simulink model "Speed_Density"  (R2025b)
settings: Solver=VariableStepAuto  StartTime=0.0  StopTime=10.0  RelTol=1e-3
model workspace (MAT data in the model file):
  P0 = 1
  R_EGR = 1
  T0 = 1
  d0 = 1
  nv = 1
settings Model: Creator=Pai  LastModifiedBy=Pai

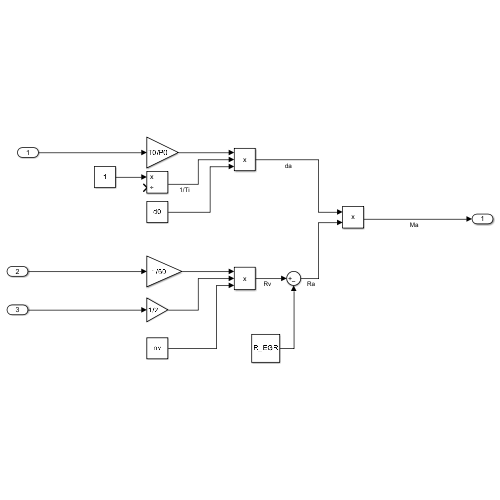
[thumbnail: Simulink's stored preview of the top-level diagram]
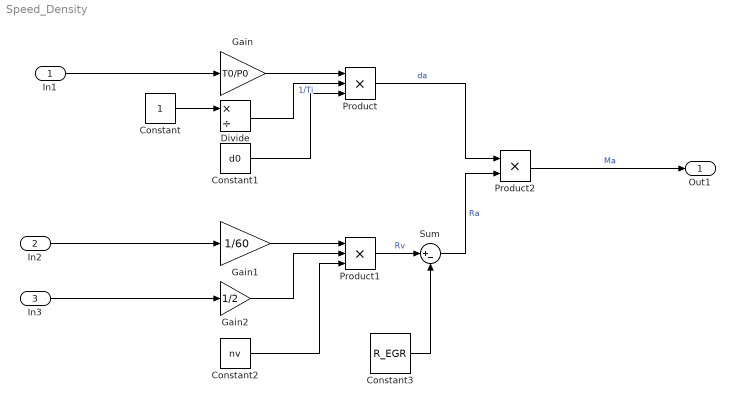
== system Speed_Density ==
  In1 : Inport
  In2 : Inport  Port=2
  In3 : Inport  Port=3
  Constant : Constant
  Constant1 : Constant  Value=d0
  Constant2 : Constant  Value=nv
  Constant3 : Constant  Value=R_EGR
  Divide : Product  Inputs=*/
  Gain : Gain  Gain=T0/P0
  Gain1 : Gain  Gain=1/60
  Gain2 : Gain  Gain=1/2
  Product : Product  Inputs=3
  Product1 : Product  Inputs=3
  Product2 : Product
  Sum : Sum  Inputs=|+-
  Out1 : Outport
  wires:
  Constant/1 -> Divide/1
  Divide/1 -> Product/2  "1/Ti"
  Gain/1 -> Product/1
  Constant1/1 -> Product/3
  Gain1/1 -> Product1/1
  Gain2/1 -> Product1/2
  Constant2/1 -> Product1/3
  Constant3/1 -> Sum/2
  Product1/1 -> Sum/1  "Rv"
  Product/1 -> Product2/1  "da"
  Sum/1 -> Product2/2  "Ra"
  In1/1 -> Gain/1
  In2/1 -> Gain1/1
  In3/1 -> Gain2/1
  Product2/1 -> Out1/1  "Ma"
